simulink model "MPCmodel"  (R2022b)
settings: Solver=VariableStepAuto  StartTime=0.0  StopTime=t_ref(end)  RelTol=1e-3
values from neighbouring files (symbols this model uses):
  A = [-0.806016499045  0  0; 0  -0.259988578457  0; 0  0  -1.03426188577]    [StateSpace.mat]
  B_mod = B(1:3,1:3)    [MPCData.m]
  C = eye(3)    [MPCData.m]    (also in StateSpace.mat = [1  0  0; 0  1  0; 0  0  1])
  D_mod = B(1:3,4:end)    [MPCData.m]
libraries: mpclib x1
settings Model: Creator=hp  LastModifiedBy=hp

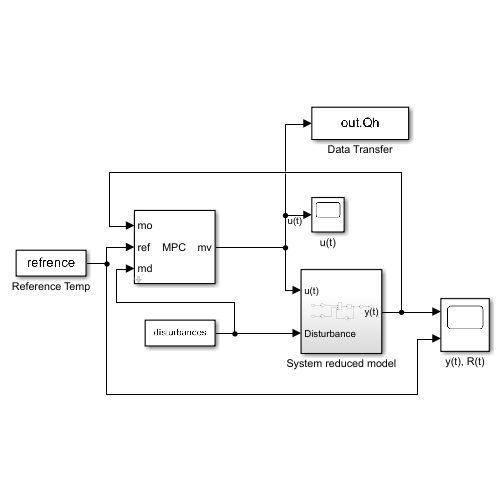
[thumbnail: Simulink's stored preview of the top-level diagram]
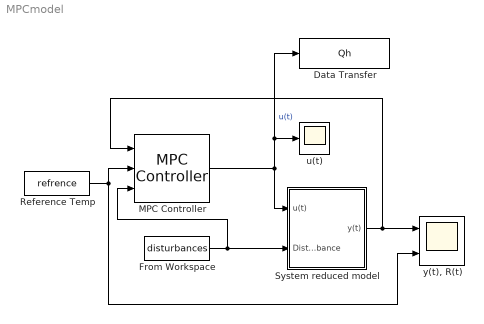
== system MPCmodel ==
  Data Transfer : ToWorkspace  VariableName=Qh  SaveFormat=Timeseries  SampleTime=-1
  From Workspace : FromWorkspace  VariableName=disturbances
  MPC Controller : mpclib/MPC Controller  SCDEnableBlockLinearizationSpecification=on  mpcobj=MPCobj  is_multiple=0  enable_value=0  return_u0=off  updateMPCinCallerWorkspace=on  md_inport=on  mv_inport=off  uref_inport=off  return_cost=off  return_mvseq=off  return_qpstatus=off  return_xseq=off  return_state=off  return_ovseq=off  state_inport=off  umin_inport=off  umax_inport=off  ymin_inport=off  ymax_inport=off  cc_inport=off  ywt_inport=off  uwt_inport=off  duwt_inport=off  rhoeps_inport=off  pm_inport=off  MaximumP=10  HorizonChoice=FixedHorizon  n_ts=0.25  n_p=20  n_mv=3  n_md=8  n_ud=0  n_mo=3  n_uo=0  BlockDataType=double  SampleTimeInherited=off  switch_inport=off
  Reference Temp : FromWorkspace  VariableName=refrence  SampleTime=0.25
  System reduced model : Subsystem
  u(t) : Scope
  "y(t), R(t)" : Scope  NumInputPorts=2
  wires:
  MPC Controller/1 -> Data Transfer/1, u(t)/1, System reduced model/1(u(t))  "u(t)"
  System reduced model/1(y(t)) -> MPC Controller/1, "y(t), R(t)"/1
  Reference Temp/1 -> MPC Controller/2, "y(t), R(t)"/2
  From Workspace/1 -> MPC Controller/3, System reduced model/2(Disturbance)

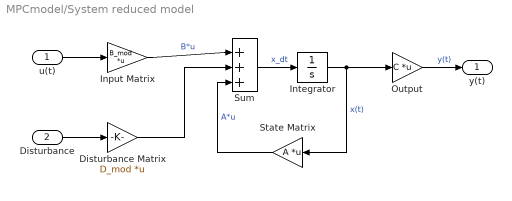
== system MPCmodel/System reduced model ==
  u(t) : Inport
  Disturbance : Inport  Port=2
  Disturbance Matrix : Gain  Gain=D_mod  Multiplication=Matrix(K*u)
  Input Matrix : Gain  Gain=B_mod  Multiplication=Matrix(K*u)
  Integrator : Integrator
  Output : Gain  Gain=C  Multiplication=Matrix(K*u)
  State Matrix : Gain  Gain=A  Multiplication=Matrix(K*u)
  Sum : Sum  Inputs=|+++
  y(t) : Outport
  wires:
  Integrator/1 -> Output/1, State Matrix/1  "x(t)"
  Input Matrix/1 -> Sum/1  "B*u"
  Sum/1 -> Integrator/1  "x_dt"
  State Matrix/1 -> Sum/3  "A*u"
  Output/1 -> y(t)/1  "y(t)"
  u(t)/1 -> Input Matrix/1
  Disturbance/1 -> Disturbance Matrix/1
  Disturbance Matrix/1 -> Sum/2
